simulink model "Non_ideal"  (R2025b)
settings: Solver=VariableStepAuto  StartTime=0.0  StopTime=4.6  RelTol=1e-3
values from neighbouring files (symbols this model uses):
  A0 = 1/w    (= 7.8125e-09)    [init.m]
  a1 = a(1)    [init.m]
  a2 = a(2)    [init.m]
  a3 = a(3)    [init.m]
  a4 = a(4)    [init.m]
  A_flick = 1e-9    (= 1e-09)    [init.m]
  Ain = 1.8    [init.m]
  Amax = 1.8    [init.m]
  b1 = b(1)    [init.m]
  c1 = c(1)    [init.m]
  c2 = c(2)    [init.m]
  c3 = c(3)    [init.m]
  c4 = c(4)    [init.m]
  fin = 250    [init.m]
  fir_coefficients = firpm(MaxTaps-1, F, A, W)    [fir_coeff.m]
  fs = 128e3    (= 128000)    [init.m]
  fsr = (2*pi)*fs*1.8    (= 1447645.89477)    [init.m]
  g1 = g(1)    [init.m]
  g2 = g(2)    [init.m]
  Gj = 1e5    (= 100000)    [init.m]
  h = h / max(h)    [cic_comp_coeff_calc.m]    (also in gain_calculate.m = tf.k * evalRP(tf.zeros,z) ./ evalRP(tf.poles,z))
  halfband_coeff = firhalfband(N, kaiser(N+1, beta))    [fir_halfband_coeff.m]
  j_rms = 0.3    [init.m]
  scale = 1.6    [init.m]
  w = (2*(1:order)'-1)*pi/order    [gain_calculate.m]    (also in init.m = 128000000)
libraries: dsphdlfiltering2 x4, dspsigops x2, dspfdesign x1
settings Model: Creator=sohom  LastModifiedBy=dhruv

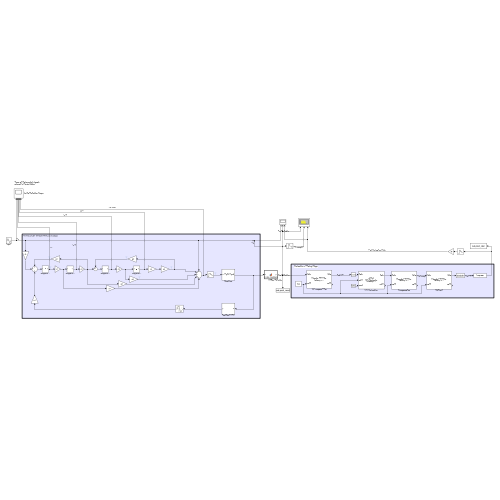
[thumbnail: Simulink's stored preview of the top-level diagram]
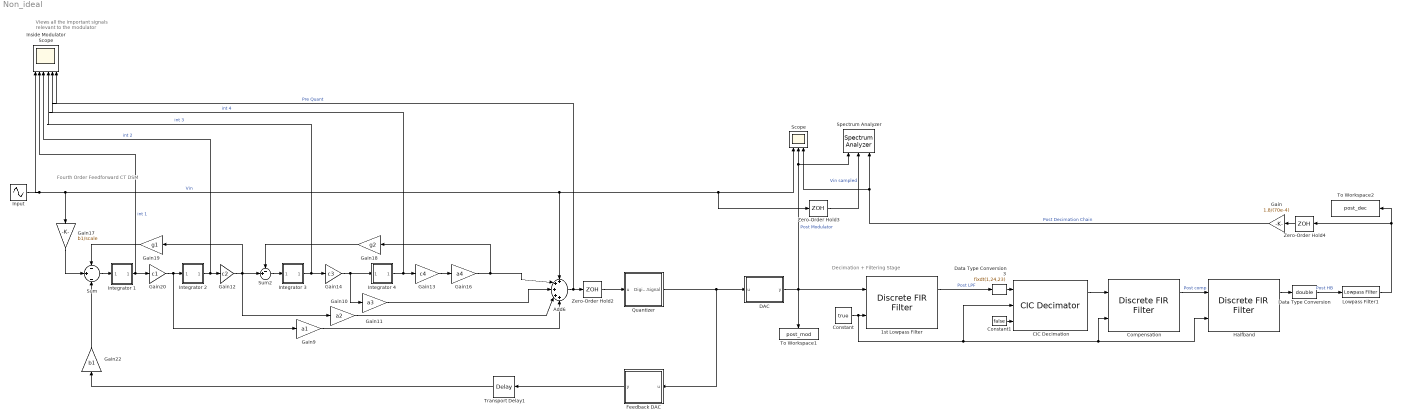
== system Non_ideal ==
  note: Fourth Order Feedforward CT DSM
  note: Views all the important signals
      | relevant to the modulator
  note: Decimation + Filtering Stage
  1st Lowpass Filter : dsphdlfiltering2/Discrete FIR Filter  NumeratorSource=Property  Numerator=[fir_coefficients]  NumeratorPrototype=[]  FilterStructure=Direct form systolic  SerializationOption=Minimum number of cycles between valid input samples  NumCycles=2  NumberOfMultipliers=2  SimulateUsing=Code generation  roundingMode=Floor  overflowMode=off  CoefficientsDataTypeStr=Inherit: Same word length as input  ResetInputPort=off  HDLGlobalReset=off  CoeffMultiplier=Multiplier  UseMultForPow2Coeff=on  FrameInputSymmOptim=on
  Add6 : Sum  Inputs=+++++
  CIC Decimation : dsphdlfiltering2/CIC Decimator  DecimationSource=Property  DecimationFactor=32  MaxDecimationFactor=2  DifferentialDelay=1  NumSections=5  GainCorrection=on  SimulateUsing=Code generation  OutputDataType=Full precision  OutputWordLength=16  ResetInputPort=on  HDLGlobalReset=off
  Compensation : dsphdlfiltering2/Discrete FIR Filter  NumeratorSource=Property  Numerator=[h]  NumeratorPrototype=[]  FilterStructure=Direct form systolic  SerializationOption=Minimum number of cycles between valid input samples  NumCycles=2  NumberOfMultipliers=2  SimulateUsing=Code generation  roundingMode=Floor  overflowMode=off  CoefficientsDataTypeStr=Inherit: Same word length as input  ResetInputPort=off  HDLGlobalReset=off  CoeffMultiplier=Multiplier  UseMultForPow2Coeff=on  FrameInputSymmOptim=on
  Constant : Constant  Value=true
  Constant1 : Constant  Value=false
  DAC : MATLAB Function  TreatAsAtomicUnit=on
  Data Type Conversion : DataTypeConversion  OutDataTypeStr=double  RndMeth=Nearest  SaturateOnIntegerOverflow=off
  Data Type Conversion3 : DataTypeConversion  OutDataTypeStr=fixdt(1,24,23)  RndMeth=Nearest  SaturateOnIntegerOverflow=off
  Feedback DAC : Subsystem
  Gain : Gain  Gain=1.8/(70e-4)
  Gain10 : Gain  Gain=a2
  Gain11 : Gain  Gain=a3
  Gain12 : Gain  Gain=c2
  Gain13 : Gain  Gain=c4
  Gain14 : Gain  Gain=c3
  Gain16 : Gain  Gain=a4
  Gain17 : Gain  Gain=b1/scale
  Gain18 : Gain  Gain=g2
  Gain19 : Gain  Gain=g1
  Gain20 : Gain  Gain=c1
  Gain22 : Gain  Gain=b1
  Gain9 : Gain  Gain=a1
  Halfband : dsphdlfiltering2/Discrete FIR Filter  NumeratorSource=Property  Numerator=[halfband_coeff]  NumeratorPrototype=[]  FilterStructure=Direct form systolic  SerializationOption=Minimum number of cycles between valid input samples  NumCycles=2  NumberOfMultipliers=2  SimulateUsing=Code generation  roundingMode=Floor  overflowMode=off  CoefficientsDataTypeStr=Inherit: Same word length as input  ResetInputPort=off  HDLGlobalReset=off  CoeffMultiplier=Multiplier  UseMultForPow2Coeff=on  FrameInputSymmOptim=on
  Input : Sin  Amplitude=Ain  Frequency=2*pi*fin  SampleTime=0
  Inside Modulator Scope : Scope  NumInputPorts=6
      settings: ActiveDisplayYMinimum=-1  ActiveDisplayYMaximum=1  DataLoggingVariableName=ScopeData2
  Integrator 1 : Subsystem
      mask Display: image('download.png');
  Integrator 2 : Subsystem
      mask Display: image('download.png');
  Integrator 3 : Subsystem
      mask Display: image('download.png');
  Integrator 4 : Subsystem
      mask Display: image('download.png');
  Lowpass Filter1 : dspfdesign/Lowpass Filter  FilterType=FIR  DesignForMinimumOrder=on  FilterOrder=50  PassbandFrequency=1000  StopbandFrequency=2000  PassbandRipple=0.01  StopbandAttenuation=80  SampleRateMode=Specify on dialog  SampleRate=fs  SimulateUsing=Interpreted execution  roundingMode=Floor  coeffsDataTypeStr=fixdt(1,16)
  Quantizer : Subsystem
  Scope : Scope  NumInputPorts=3
      settings: ActiveDisplayYMinimum=-2.2360659087505561  ActiveDisplayYMaximum=2.257708308181404
  Spectrum Analyzer : SpectrumAnalyzer  NumInputPorts=3  WindowPosition=[0.000000,36.000000,1920.000000,1009.000000,]  ScopeFrameLocation=window  SampleRate=44.1e3  PlotAsTwoSidedSpectrum=off  WindowInvariantSamplesPerUpdate=on  FrequencySpan=Start and stop frequencies  StartFrequency=20  StopFrequency=20e3  YLimits=[NaN NaN]  ShowLegend=on  SelectedToolstripTab=spectrumAnalyzerToolstrip.measurementsTab
  Sum : Sum  Inputs=-|+|-
  Sum2 : Sum  Inputs=-+|
  To Workspace1 : ToWorkspace  VariableName=post_mod  SaveFormat=Timeseries  SampleTime=-1
  To Workspace2 : ToWorkspace  VariableName=post_dec  SaveFormat=Timeseries  SampleTime=-1
  Transport Delay1 : TransportDelay  DelayTime=0.1/fs
  Zero-Order Hold2 : ZeroOrderHold  SampleTime=1/fs
  Zero-Order Hold3 : ZeroOrderHold  SampleTime=1/fs
  Zero-Order Hold4 : ZeroOrderHold  SampleTime=1/fs
  wires:
  Gain11/1 -> Add6/3
  Gain10/1 -> Add6/4
  Gain17/1 -> Sum/2
  Gain22/1 -> Sum/3
  Gain19/1 -> Sum/1
  Gain16/1 -> Gain18/1, Add6/2
  Transport Delay1/1 -> Gain22/1
  Gain9/1 -> Add6/5
  Gain18/1 -> Sum2/1
  Gain12/1 -> Gain19/1, Sum2/2, Gain10/1
  Gain20/1 -> Integrator 2/1(Input), Gain9/1
  Gain14/1 -> Integrator 4/1(Input), Gain11/1
  Quantizer/1(Digital Signal) -> Feedback DAC/1(u), DAC/1(u)
  Zero-Order Hold2/1 -> Quantizer/1(u)
  Feedback DAC/1(y) -> Transport Delay1/1
  Sum/1 -> Integrator 1/1(Input)
  Sum2/1 -> Integrator 3/1(Input)
  Integrator 2/1(Output) -> Inside Modulator Scope/3, Gain12/1  "int 2"
  Integrator 4/1(Output) -> Gain13/1, Inside Modulator Scope/5  "int 4"
  Integrator 1/1(Output) -> Gain20/1, Inside Modulator Scope/2  "int 1"
  Add6/1 -> Inside Modulator Scope/6, Zero-Order Hold2/1  "Pre Quant"
  Integrator 3/1(Output) -> Inside Modulator Scope/4, Gain14/1  "int 3"
  Data Type Conversion/1 -> Lowpass Filter1/1  "Post HB"
  Compensation/1 -> Halfband/1  "Post comp"
  CIC Decimation/1 -> Compensation/1
  Zero-Order Hold4/1 -> Gain/1
  Halfband/1 -> Data Type Conversion/1
  Constant1/1 -> CIC Decimation/3
  DAC/1(y) -> Spectrum Analyzer/1, Scope/2, To Workspace1/1, 1st Lowpass Filter/1  "Post Modulator"
  Input/1 -> Inside Modulator Scope/1, Gain17/1, Zero-Order Hold3/1, Scope/1, Add6/1  "Vin"
  1st Lowpass Filter/1 -> Data Type Conversion3/1  "Post LPF"
  Lowpass Filter1/1 -> To Workspace2/1, Zero-Order Hold4/1
  Constant/1 -> CIC Decimation/2, Halfband/2, Compensation/2, 1st Lowpass Filter/2
  Zero-Order Hold3/1 -> Spectrum Analyzer/2  "Vin sampled"
  Data Type Conversion3/1 -> CIC Decimation/1
  Gain/1 -> Scope/3, Spectrum Analyzer/3  "Post Decimation Chain"
  Gain13/1 -> Gain16/1

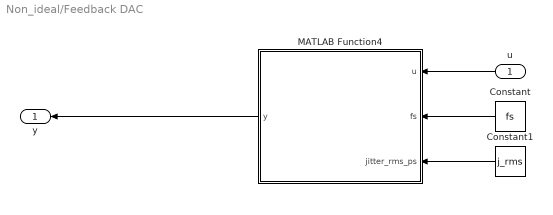
== system Non_ideal/Feedback DAC ==
  u : Inport
  Constant : Constant  Value=fs
  Constant1 : Constant  Value=j_rms
  MATLAB Function4 : MATLAB Function  TreatAsAtomicUnit=on
  y : Outport
  wires:
  MATLAB Function4/1(y) -> y/1
  Constant1/1 -> MATLAB Function4/3(jitter_rms_ps)
  Constant/1 -> MATLAB Function4/2(fs)
  u/1 -> MATLAB Function4/1(u)

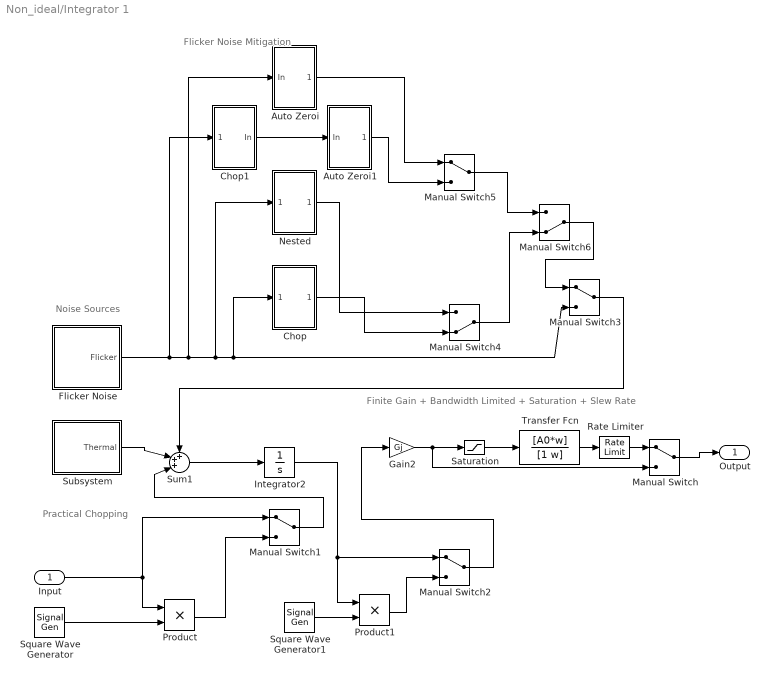
== system Non_ideal/Integrator 1 ==
  note: Finite Gain + Bandwidth Limited + Saturation + Slew Rate
  note: Flicker Noise Mitigation
  note: Practical Chopping
  note: Noise Sources
  Input : Inport
  Auto Zeroi : Subsystem
  Auto Zeroi1 : Subsystem
  Chop : Subsystem
  Chop1 : Subsystem
  Flicker Noise : Subsystem
  Gain2 : Gain  Gain=Gj
  Integrator2 : Integrator
  Manual Switch{,1..3,5} (5 alike) : ManualSwitch
  Manual Switch4 : ManualSwitch  CurrentSetting=0
  Manual Switch6 : ManualSwitch  CurrentSetting=0
  Nested : Subsystem
  Product : Product
  Product1 : Product
  Rate Limiter : RateLimiter  RisingSlewLimit=fsr  FallingSlewLimit=-fsr  SampleTimeMode=inherited
  Saturation : Saturate  UpperLimit=Amax  LowerLimit=-Amax
  Square Wave Generator : SignalGenerator  WaveForm=square  Frequency=8000
  Square Wave Generator1 : SignalGenerator  WaveForm=square  Frequency=8000
  Subsystem : Subsystem
  Sum1 : Sum  Inputs=+++|
  Transfer Fcn : TransferFcn  Numerator=[A0*w]  Denominator=[1 w]
  Output : Outport
  wires:
  Subsystem/1(Thermal) -> Sum1/2
  Manual Switch/1 -> Output/1
  Sum1/1 -> Integrator2/1
  Rate Limiter/1 -> Manual Switch/1
  Transfer Fcn/1 -> Rate Limiter/1
  Gain2/1 -> Manual Switch/2, Saturation/1
  Saturation/1 -> Transfer Fcn/1
  Square Wave Generator/1 -> Product/2
  Product/1 -> Manual Switch1/2
  Input/1 -> Manual Switch1/1, Product/1
  Product1/1 -> Manual Switch2/2
  Integrator2/1 -> Manual Switch2/1, Product1/1
  Square Wave Generator1/1 -> Product1/2
  Manual Switch2/1 -> Gain2/1
  Manual Switch1/1 -> Sum1/3
  Flicker Noise/1(Flicker) -> Chop1/1(Flicker), Auto Zeroi/1(In), Chop/1(Flicker), Manual Switch3/2, Nested/1(In1)
  Manual Switch3/1 -> Sum1/1
  Auto Zeroi/1(Out1) -> Manual Switch5/1
  Chop/1(Out1) -> Manual Switch4/2
  Nested/1(Out1) -> Manual Switch4/1
  Manual Switch4/1 -> Manual Switch6/2
  Manual Switch6/1 -> Manual Switch3/1
  Chop1/1(In) -> Auto Zeroi1/1(In)
  Auto Zeroi1/1(Out1) -> Manual Switch5/2
  Manual Switch5/1 -> Manual Switch6/1

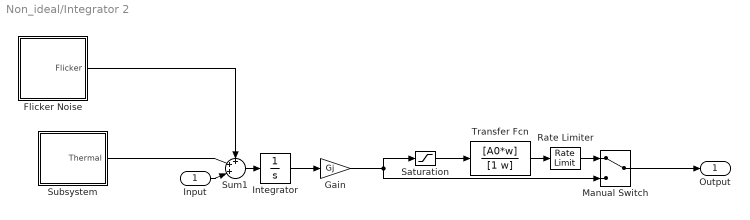
== system Non_ideal/Integrator 2 ==
  Input : Inport
  Flicker Noise : Subsystem
  Gain : Gain  Gain=Gj
  Integrator : Integrator
  Manual Switch : ManualSwitch
  Rate Limiter : RateLimiter  RisingSlewLimit=fsr  FallingSlewLimit=-fsr  SampleTimeMode=inherited
  Saturation : Saturate  UpperLimit=Amax  LowerLimit=-Amax
  Subsystem : Subsystem
  Sum1 : Sum  Inputs=+++|
  Transfer Fcn : TransferFcn  Numerator=[A0*w]  Denominator=[1 w]
  Output : Outport
  wires:
  Input/1 -> Sum1/3
  Subsystem/1(Thermal) -> Sum1/2
  Flicker Noise/1(Flicker) -> Sum1/1
  Manual Switch/1 -> Output/1
  Sum1/1 -> Integrator/1
  Integrator/1 -> Gain/1
  Rate Limiter/1 -> Manual Switch/1
  Transfer Fcn/1 -> Rate Limiter/1
  Gain/1 -> Manual Switch/2, Saturation/1
  Saturation/1 -> Transfer Fcn/1

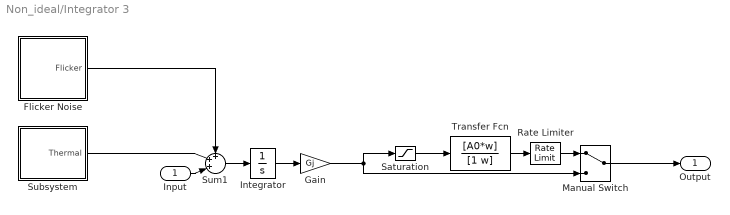
== system Non_ideal/Integrator 3 ==
  Input : Inport
  Flicker Noise : Subsystem
  Gain : Gain  Gain=Gj
  Integrator : Integrator
  Manual Switch : ManualSwitch
  Rate Limiter : RateLimiter  RisingSlewLimit=fsr  FallingSlewLimit=-fsr  SampleTimeMode=inherited
  Saturation : Saturate  UpperLimit=Amax  LowerLimit=-Amax
  Subsystem : Subsystem
  Sum1 : Sum  Inputs=+++|
  Transfer Fcn : TransferFcn  Numerator=[A0*w]  Denominator=[1 w]
  Output : Outport
  wires:
  Input/1 -> Sum1/3
  Subsystem/1(Thermal) -> Sum1/2
  Flicker Noise/1(Flicker) -> Sum1/1
  Manual Switch/1 -> Output/1
  Sum1/1 -> Integrator/1
  Integrator/1 -> Gain/1
  Rate Limiter/1 -> Manual Switch/1
  Transfer Fcn/1 -> Rate Limiter/1
  Gain/1 -> Manual Switch/2, Saturation/1
  Saturation/1 -> Transfer Fcn/1

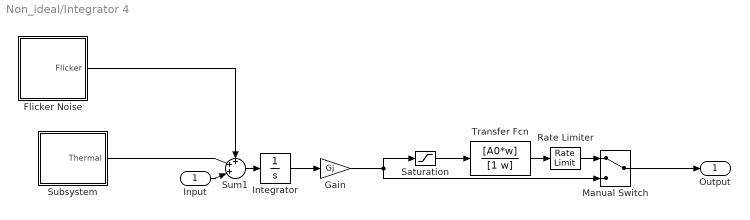
== system Non_ideal/Integrator 4 ==
  Input : Inport
  Flicker Noise : Subsystem
  Gain : Gain  Gain=Gj
  Integrator : Integrator
  Manual Switch : ManualSwitch
  Rate Limiter : RateLimiter  RisingSlewLimit=fsr  FallingSlewLimit=-fsr  SampleTimeMode=inherited
  Saturation : Saturate  UpperLimit=Amax  LowerLimit=-Amax
  Subsystem : Subsystem
  Sum1 : Sum  Inputs=+++|
  Transfer Fcn : TransferFcn  Numerator=[A0*w]  Denominator=[1 w]
  Output : Outport
  wires:
  Input/1 -> Sum1/3
  Subsystem/1(Thermal) -> Sum1/2
  Flicker Noise/1(Flicker) -> Sum1/1
  Manual Switch/1 -> Output/1
  Sum1/1 -> Integrator/1
  Integrator/1 -> Gain/1
  Rate Limiter/1 -> Manual Switch/1
  Transfer Fcn/1 -> Rate Limiter/1
  Gain/1 -> Manual Switch/2, Saturation/1
  Saturation/1 -> Transfer Fcn/1

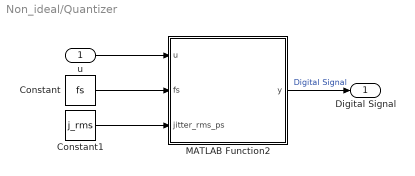
== system Non_ideal/Quantizer ==
  u : Inport
  Constant : Constant  Value=fs
  Constant1 : Constant  Value=j_rms
  MATLAB Function2 : MATLAB Function  TreatAsAtomicUnit=on
  Digital Signal : Outport
  wires:
  MATLAB Function2/1(y) -> Digital Signal/1  "Digital Signal"
  u/1 -> MATLAB Function2/1(u)
  Constant1/1 -> MATLAB Function2/3(jitter_rms_ps)
  Constant/1 -> MATLAB Function2/2(fs)

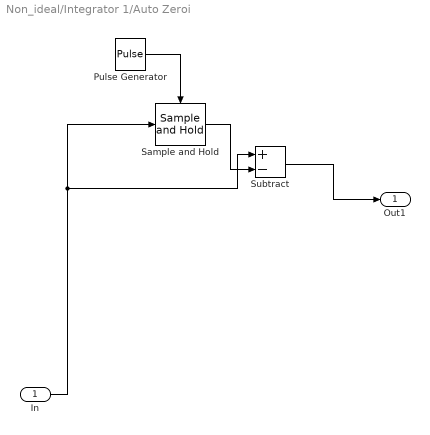
== system Non_ideal/Integrator 1/Auto Zeroi ==
  In : Inport
  Pulse Generator : DiscretePulseGenerator  PulseType=Time based  Period=10/128000
  Sample and Hold : dspsigops/Sample and Hold  trig=Rising edge  initCond=0  latchinput=off
  Subtract : Sum  Inputs=+-
  Out1 : Outport
  wires:
  Subtract/1 -> Out1/1
  Pulse Generator/1 -> Sample and Hold/Trigger
  In/1 -> Subtract/1, Sample and Hold/1
  Sample and Hold/1 -> Subtract/2

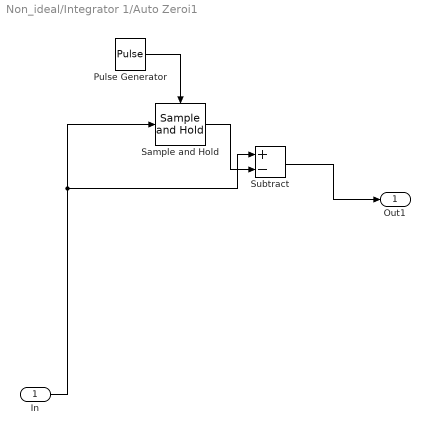
== system Non_ideal/Integrator 1/Auto Zeroi1 ==
  In : Inport
  Pulse Generator : DiscretePulseGenerator  PulseType=Time based  Period=10/128000
  Sample and Hold : dspsigops/Sample and Hold  trig=Rising edge  initCond=0  latchinput=off
  Subtract : Sum  Inputs=+-
  Out1 : Outport
  wires:
  Subtract/1 -> Out1/1
  Pulse Generator/1 -> Sample and Hold/Trigger
  In/1 -> Subtract/1, Sample and Hold/1
  Sample and Hold/1 -> Subtract/2

== system Non_ideal/Integrator 1/Chop ==
  Flicker : Inport
  Product3 : Product
  Square Wave Generator3 : SignalGenerator  WaveForm=square  Frequency=32000
  Out1 : Outport
  wires:
  Product3/1 -> Out1/1
  Square Wave Generator3/1 -> Product3/2
  Flicker/1 -> Product3/1

== system Non_ideal/Integrator 1/Chop1 ==
  Flicker : Inport
  Product3 : Product
  Square Wave Generator3 : SignalGenerator  WaveForm=square  Frequency=32000
  In : Outport
  wires:
  Product3/1 -> In/1
  Square Wave Generator3/1 -> Product3/2
  Flicker/1 -> Product3/1

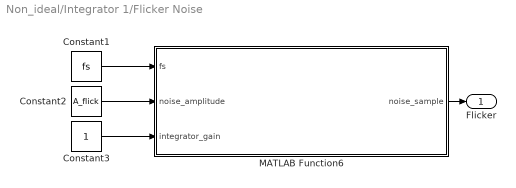
== system Non_ideal/Integrator 1/Flicker Noise ==
  Constant1 : Constant  Value=fs
  Constant2 : Constant  Value=A_flick
  Constant3 : Constant
  MATLAB Function6 : MATLAB Function  TreatAsAtomicUnit=on
  Flicker : Outport
  wires:
  Constant2/1 -> MATLAB Function6/2(noise_amplitude)
  Constant3/1 -> MATLAB Function6/3(integrator_gain)
  Constant1/1 -> MATLAB Function6/1(fs)
  MATLAB Function6/1(noise_sample) -> Flicker/1

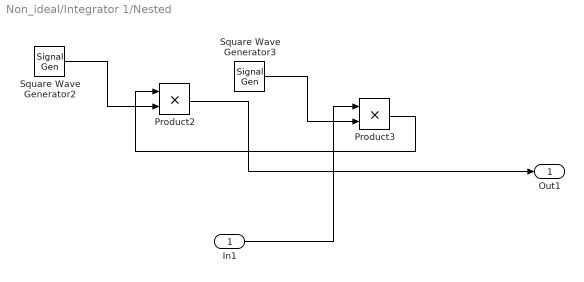
== system Non_ideal/Integrator 1/Nested ==
  In1 : Inport
  Product2 : Product
  Product3 : Product
  Square Wave Generator2 : SignalGenerator  WaveForm=square  Frequency=4000
  Square Wave Generator3 : SignalGenerator  WaveForm=square  Frequency=32000
  Out1 : Outport
  wires:
  Product2/1 -> Out1/1
  Square Wave Generator3/1 -> Product3/2
  Product3/1 -> Product2/1
  In1/1 -> Product3/1
  Square Wave Generator2/1 -> Product2/2

== system Non_ideal/Integrator 1/Subsystem ==
  Constant1 : Constant  Value=fs
  MATLAB Function6 : MATLAB Function  TreatAsAtomicUnit=on
  Thermal : Outport
  wires:
  Constant1/1 -> MATLAB Function6/1(fs)
  MATLAB Function6/1(noise_out) -> Thermal/1

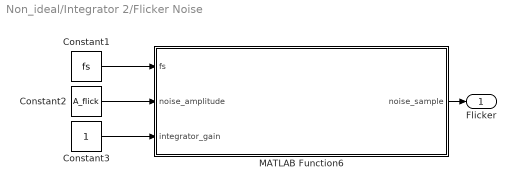
== system Non_ideal/Integrator 2/Flicker Noise ==
  Constant1 : Constant  Value=fs
  Constant2 : Constant  Value=A_flick
  Constant3 : Constant
  MATLAB Function6 : MATLAB Function  TreatAsAtomicUnit=on
  Flicker : Outport
  wires:
  Constant2/1 -> MATLAB Function6/2(noise_amplitude)
  Constant3/1 -> MATLAB Function6/3(integrator_gain)
  Constant1/1 -> MATLAB Function6/1(fs)
  MATLAB Function6/1(noise_sample) -> Flicker/1

== system Non_ideal/Integrator 2/Subsystem ==
  Constant1 : Constant  Value=fs
  MATLAB Function6 : MATLAB Function  TreatAsAtomicUnit=on
  Thermal : Outport
  wires:
  Constant1/1 -> MATLAB Function6/1(fs)
  MATLAB Function6/1(noise_out) -> Thermal/1

== system Non_ideal/Integrator 3/Flicker Noise ==
  Constant1 : Constant  Value=fs
  Constant2 : Constant  Value=A_flick
  Constant3 : Constant
  MATLAB Function6 : MATLAB Function  TreatAsAtomicUnit=on
  Flicker : Outport
  wires:
  Constant2/1 -> MATLAB Function6/2(noise_amplitude)
  Constant3/1 -> MATLAB Function6/3(integrator_gain)
  Constant1/1 -> MATLAB Function6/1(fs)
  MATLAB Function6/1(noise_sample) -> Flicker/1

== system Non_ideal/Integrator 3/Subsystem ==
  Constant1 : Constant  Value=fs
  MATLAB Function6 : MATLAB Function  TreatAsAtomicUnit=on
  Thermal : Outport
  wires:
  Constant1/1 -> MATLAB Function6/1(fs)
  MATLAB Function6/1(noise_out) -> Thermal/1

== system Non_ideal/Integrator 4/Flicker Noise ==
  Constant1 : Constant  Value=fs
  Constant2 : Constant  Value=A_flick
  Constant3 : Constant
  MATLAB Function6 : MATLAB Function  TreatAsAtomicUnit=on
  Flicker : Outport
  wires:
  Constant2/1 -> MATLAB Function6/2(noise_amplitude)
  Constant3/1 -> MATLAB Function6/3(integrator_gain)
  Constant1/1 -> MATLAB Function6/1(fs)
  MATLAB Function6/1(noise_sample) -> Flicker/1

== system Non_ideal/Integrator 4/Subsystem ==
  Constant1 : Constant  Value=fs
  MATLAB Function6 : MATLAB Function  TreatAsAtomicUnit=on
  Thermal : Outport
  wires:
  Constant1/1 -> MATLAB Function6/1(fs)
  MATLAB Function6/1(noise_out) -> Thermal/1

== matlab function Non_ideal/Integrator 2/Flicker Noise/MATLAB Function6 ==
  data: noise_sample output; fs input; noise_amplitude input; integrator_gain input
function noise_sample = flicker_noise_stream(fs, noise_amplitude, integrator_gain)
% 1/f Flicker Noise Generator for CTDSM
% Paste this entire function into Simulink MATLAB Function block
%
% Inputs:
%   fs               - Sampling frequency (Hz)
%   noise_amplitude  - Noise amplitude (V/sqrt(Hz) at 1Hz), e.g., 1e-7
%   integrator_gain  - Integrator coefficient, e.g., 1.0
%
% Output:
%   noise_sample     - Single noise sample for this time step

persistent generators counters num_gen

% Initialize on first call
if isempty(generators)
    num_gen = 16;
    generators = randn(num_gen, 1);
    counters = zeros(num_gen, 1);
end

% Generate 1/f noise using Voss-McCartney algorithm
noise_sample = 0;
for k = 1:num_gen
    counters(k) = counters(k) + 1;
    update_rate = 2^k;
    
    % Update generator when counter reaches update rate
    if counters(k) >= update_rate
        generators(k) = randn();
        counters(k) = 0;
    end
    
    noise_sample = noise_sample + generators(k);
end

% Normalize and scale
noise_sample = noise_sample / sqrt(num_gen);

% Scale with signal bandwidth (0.25 to 1 kHz)
signal_bw = 1000;
noise_sample = noise_sample * sqrt(signal_bw);

% Apply user-specified amplitude
noise_sample = noise_sample * noise_amplitude;

% Scale by integrator characteristics
noise_sample = noise_sample * sqrt(abs(integrator_gain));

% Convert from PSD to time-domain amplitude
noise_sample = noise_sample * sqrt(fs/2);

end

== matlab function Non_ideal/Integrator 1/Flicker Noise/MATLAB Function6 ==
  data: noise_sample output; fs input; noise_amplitude input; integrator_gain input
function noise_sample = flicker_noise_stream(fs, noise_amplitude, integrator_gain)
% 1/f Flicker Noise Generator for CTDSM
% Paste this entire function into Simulink MATLAB Function block
%
% Inputs:
%   fs               - Sampling frequency (Hz)
%   noise_amplitude  - Noise amplitude (V/sqrt(Hz) at 1Hz), e.g., 1e-7
%   integrator_gain  - Integrator coefficient, e.g., 1.0
%
% Output:
%   noise_sample     - Single noise sample for this time step

persistent generators counters num_gen

% Initialize on first call
if isempty(generators)
    num_gen = 16;
    generators = randn(num_gen, 1);
    counters = zeros(num_gen, 1);
end

% Generate 1/f noise using Voss-McCartney algorithm
noise_sample = 0;
for k = 1:num_gen
    counters(k) = counters(k) + 1;
    update_rate = 2^k;
    
    % Update generator when counter reaches update rate
    if counters(k) >= update_rate
        generators(k) = randn();
        counters(k) = 0;
    end
    
    noise_sample = noise_sample + generators(k);
end

% Normalize and scale
noise_sample = noise_sample / sqrt(num_gen);

% Scale with signal bandwidth (0.25 to 1 kHz)
signal_bw = 1000;
noise_sample = noise_sample * sqrt(signal_bw);

% Apply user-specified amplitude
noise_sample = noise_sample * noise_amplitude;

% Scale by integrator characteristics
noise_sample = noise_sample * sqrt(abs(integrator_gain));

% Convert from PSD to time-domain amplitude
noise_sample = noise_sample * sqrt(fs/2);

end

== matlab function Non_ideal/Quantizer/MATLAB Function2 ==
  data: u input; y output; fs input; jitter_rms_ps input
function y = ct_quantizer(u, fs, jitter_rms_ps)
% CT DSM Quantizer with Clock Jitter and Thermometer Code Output
% Insert this as a MATLAB Function block in Simulink
%
% INPUTS:
%   u              - Input signal from loop filter
%   fs             - Sampling frequency (Hz)
%   jitter_rms_ps  - RMS clock jitter in picoseconds (ps)
%                    Set to 0 for ideal case (no jitter)
%
% PARAMETERS (modify these at the top)
% =========================================================================
N_LEVELS = 16;           % Number of quantization levels (1-bit = 2 levels)
INPUT_MIN = -1.8;        % Minimum input range (V)
INPUT_MAX = 1.8;         % Maximum input range (V)

% PERSISTENT VARIABLES - MUST BE DECLARED AT TOP!
% =========================================================================
persistent u_prev;

% JITTER GUIDELINES (typical values for different applications):
% =========================================================================
% Ultra-low jitter (< 100 fs):   20+ bit ENOB, high-end audio/instrumentation
% Low jitter (100 fs - 1 ps):    18-20 bit ENOB, precision converters
% Moderate jitter (1-10 ps):     14-16 bit ENOB, general purpose ADCs
% High jitter (10-100 ps):       10-12 bit ENOB, cost-optimized designs
% Very high jitter (> 100 ps):   < 10 bit ENOB, low-performance systems
%
% For YOUR CTDSM (ENOB 16-19 target):
% RECOMMENDED: jitter_rms_ps = 0.5 to 2 ps (500 fs to 2 ps)
%
% Jitter SNR Formula: SNR_jitter(dB) = -20*log10(2*pi*f_in*σ_jitter)
% For f_in = 1 kHz, jitter = 1 ps: SNR ≈ 104 dB (17 bits)
% =========================================================================

% Validate parameters
assert(N_LEVELS >= 2, 'N_LEVELS must be at least 2');
assert(INPUT_MAX > INPUT_MIN, 'INPUT_MAX must be greater than INPUT_MIN');
assert(fs > 0, 'Sampling frequency must be positive');
assert(jitter_rms_ps >= 0, 'Jitter must be non-negative');

% Initialize persistent variable on first call
if isempty(u_prev)
    u_prev = u;
end

% Calculate jitter-induced timing error
if jitter_rms_ps > 0
    % Convert jitter from picoseconds to seconds
    jitter_rms_sec = jitter_rms_ps * 1e-12;
    
    % Generate random timing error (Gaussian distribution)
    timing_error = jitter_rms_sec * randn();
    
    % Calculate slew rate
    Ts = 1/fs;  % Sampling period
    slew_rate = (u - u_prev) / Ts;  % V/s
    
    % Calculate voltage error due to timing jitter
    % ΔV = (dV/dt) × Δt
    voltage_error = slew_rate * timing_error;
    
    % Apply jitter error to input
    u_jittered = u + voltage_error;
else
    % Ideal case: no jitter
    u_jittered = u;
end

% Update previous value for next iteration
u_prev = u;

% Input saturation (clip to range)
u_clipped = max(INPUT_MIN, min(INPUT_MAX, u_jittered));

% Mid-tread quantizer: zero is a quantization level
% For N levels, we have (N-1) thresholds
if N_LEVELS == 2
    % Special case: 1-bit quantizer
    % Threshold at 0 (mid-tread)
    if u_clipped >= 0
        quant_level = 1;  % Upper level
    else
        quant_level = 0;  % Lower level
    end
else
    % Multi-bit quantizer
    % Calculate thresholds for mid-tread configuration
    step = (INPUT_MAX - INPUT_MIN) / (N_LEVELS - 1);
    
    % Find which level the input corresponds to
    quant_level = round((u_clipped - INPUT_MIN) / step);
    
    % Ensure level is in valid range [0, N_LEVELS-1]
    quant_level = max(0, min(N_LEVELS - 1, quant_level));
end

% Convert to thermometer code
thermometer = zeros(1, N_LEVELS - 1);
for i = 1:(N_LEVELS - 1)
    if i <= quant_level
        thermometer(i) = 1;
    end
end

% Output as column vector
y = thermometer';

end

== matlab function Non_ideal/Integrator 2/Subsystem/MATLAB Function6 ==
  data: fs input; noise_out output
function noise_out = thermal_noise_circuit_based(fs)
    % Physical parameters
    T = 300;                    % Temperature (K)
    k = 1.38e-23;              % Boltzmann constant (J/K)
    
    % CIRCUIT PARAMETERS - These should come from your circuit design!
    % =================================================================
    
    % Option A: If you have op-amp specs
    % Input-referred noise voltage density (typical op-amp datasheet value)
    % Examples:
    %   - Precision op-amp: 5-10 nV/√Hz
    %   - General purpose: 10-20 nV/√Hz
    %   - Low noise: 1-5 nV/√Hz
    e_n = 10e-9;  % V/√Hz (10 nV/√Hz - typical precision op-amp)
    
    % Option B: If you have resistor values
    % Typical switched-capacitor or continuous-time integrator
    R_eq = 10e3;  % Equivalent noise resistance (10 kΩ typical)
    
    % Choose one method:
    % Method 1: Direct from op-amp noise spec
    noise_density = e_n;  % V/√Hz
    
    % Method 2: From thermal resistance
    % noise_density = sqrt(4 * k * T * R_eq);  % V/√Hz
    
    % =================================================================
    
    % Noise bandwidth (full Nyquist)
    BW = fs / 2;
    
    % Total RMS noise
    V_noise_rms = noise_density * sqrt(BW);
    
    % Generate white Gaussian noise sample
    % Scale to match power spectral density
    noise_out = V_noise_rms * randn();
    
end

== matlab function Non_ideal/Feedback DAC/MATLAB Function4 ==
  data: u input; y output; fs input; jitter_rms_ps input
function y = ct_dac_feedback(u, fs, jitter_rms_ps)
% CT DSM Feedback DAC with Clock Jitter - Converts Thermometer Code to Analog Level
% Insert this as a MATLAB Function block in Simulink
%
% INPUTS:
%   u              - Thermometer code from quantizer
%   fs             - Sampling frequency (Hz)
%   jitter_rms_ps  - RMS clock jitter in picoseconds (ps)
%                    Set to 0 for ideal case (no jitter)
%
% PARAMETERS (must match quantizer settings)
% =========================================================================
N_LEVELS = 16;           % Number of quantization levels (must match quantizer)
OUTPUT_MIN = -1.8;       % Minimum output voltage/amplitude (V)
OUTPUT_MAX = 1.8;        % Maximum output voltage/amplitude (V)

% PERSISTENT VARIABLES - MUST BE DECLARED AT TOP!
% =========================================================================
persistent y_prev;

% JITTER GUIDELINES FOR FEEDBACK DAC (MORE CRITICAL THAN QUANTIZER):
% =========================================================================
% The feedback DAC jitter is NOT noise-shaped and appears directly at input!
% DAC jitter requirements are typically 2-5x stricter than quantizer jitter.
%
% For CTDSM (ENOB 16-19 target):
% RECOMMENDED: jitter_rms_ps = 0.2 to 1 ps (200 fs to 1 ps)
% =========================================================================

% Validate parameters
assert(N_LEVELS >= 2, 'N_LEVELS must be at least 2');
assert(OUTPUT_MAX > OUTPUT_MIN, 'OUTPUT_MAX must be greater than OUTPUT_MIN');
assert(fs > 0, 'Sampling frequency must be positive');
assert(jitter_rms_ps >= 0, 'Jitter must be non-negative');

% Decode thermometer code to level
if N_LEVELS == 2
    % Special case: 1-bit (single element vector)
    level = u(1);  % 0 or 1
else
    % Multi-bit: count number of ones in thermometer code
    level = sum(u);  % Level from 0 to (N_LEVELS-1)
end

% Convert level to analog output (mid-tread)
if N_LEVELS == 2
    % 1-bit: simple bipolar mapping
    if level == 0
        y_ideal = OUTPUT_MIN;
    else
        y_ideal = OUTPUT_MAX;
    end
else
    % Multi-bit: linear mapping
    step = (OUTPUT_MAX - OUTPUT_MIN) / (N_LEVELS - 1);
    y_ideal = OUTPUT_MIN + level * step;
end

% Initialize persistent variable on first call
if isempty(y_prev)
    y_prev = y_ideal;
end

% Apply DAC clock jitter effects
if jitter_rms_ps > 0
    % Convert jitter from picoseconds to seconds
    jitter_rms_sec = jitter_rms_ps * 1e-12;
    
    % Generate random timing error (Gaussian distribution)
    timing_error = jitter_rms_sec * randn();
    
    % Calculate DAC output slew rate (how fast DAC is switching)
    Ts = 1/fs;  % Sampling period
    dac_slew_rate = (y_ideal - y_prev) / Ts;  % V/s
    
    % Voltage error due to timing jitter at DAC output
    % ΔV = (dV/dt) × Δt
    voltage_error = dac_slew_rate * timing_error;
    
    % Apply jitter error to DAC output
    y = y_ideal + voltage_error;
    
    % Optional: Add saturation to prevent unrealistic outputs
    y = max(OUTPUT_MIN, min(OUTPUT_MAX, y));
else
    % Ideal case: no jitter
    y = y_ideal;
end

% Update previous value for next iteration
y_prev = y_ideal;

end

== matlab function Non_ideal/DAC ==
  data: u input; y output
function y = ct_dac_feedback(u)
% CT DSM Feedback DAC - Converts Thermometer Code to Analog Level
% Insert this as a MATLAB Function block in Simulink
% Compatible with ct_quantizer output
%
% PARAMETERS (must match quantizer settings)
% =========================================================================
N_LEVELS = 16;           % Number of quantization levels (must match quantizer)
OUTPUT_MIN = -1.8;      % Minimum output voltage/amplitude
OUTPUT_MAX = 1.8;       % Maximum output voltage/amplitude
% =========================================================================

% Validate parameters
assert(N_LEVELS >= 2, 'N_LEVELS must be at least 2');
assert(OUTPUT_MAX > OUTPUT_MIN, 'OUTPUT_MAX must be greater than OUTPUT_MIN');

% Decode thermometer code to level
% Thermometer code has (N_LEVELS - 1) bits
% Count the number of ones to get the level
if N_LEVELS == 2
    % Special case: 1-bit (single element vector)
    % u is [0] or [1]
    level = u(1);  % 0 or 1
else
    % Multi-bit: count number of ones in thermometer code
    level = sum(u);  % This gives level from 0 to (N_LEVELS-1)
end

% Convert level to analog output (mid-tread)
% Map level [0, 1, 2, ..., N_LEVELS-1] to analog range
% For mid-tread, ensure level corresponds to actual output values
if N_LEVELS == 2
    % 1-bit: simple bipolar mapping
    % Level 0 -> OUTPUT_MIN (-1.8)
    % Level 1 -> OUTPUT_MAX (+1.8)
    if level == 0
        y = OUTPUT_MIN;
    else
        y = OUTPUT_MAX;
    end
else
    % Multi-bit: linear mapping
    % Map level to output range with mid-tread alignment
    step = (OUTPUT_MAX - OUTPUT_MIN) / (N_LEVELS - 1);
    y = OUTPUT_MIN + level * step;
end

end

% =========================================================================
% USAGE INSTRUCTIONS FOR SIMULINK:
% =========================================================================
% 1. Add a MATLAB Function block after your quantizer
% 2. Double-click the block and paste this entire code
% 3. Connect quantizer output (thermometer code) to this block's input
% 4. This block's output goes to the feedback path (summed with input)
%
% SIGNAL FLOW:
%   Input → [Σ] → Loop Filter → Quantizer → Output
%            ↑                      ↓
%            └──────── DAC ─────────┘
%
% For 2-level (1-bit):
%   Thermometer [0] → Analog output = -1.8
%   Thermometer [1] → Analog output = +1.8
%
% For 4-level (2-bit):
%   Thermometer [0 0 0] → -1.8
%   Thermometer [1 0 0] → -0.6
%   Thermometer [1 1 0] → +0.6
%   Thermometer [1 1 1] → +1.8
%
% NOTES:
% - N_LEVELS, OUTPUT_MIN, OUTPUT_MAX must match quantizer parameters
% - This is an ideal DAC (no delay, noise, or mismatch)
% - For CT-DSM, this typically runs continuously (no sample/hold needed)
% - Output is continuous-time analog signal fed back to input summer
% =========================================================================

== matlab function Non_ideal/Integrator 3/Flicker Noise/MATLAB Function6 ==
  data: noise_sample output; fs input; noise_amplitude input; integrator_gain input
function noise_sample = flicker_noise_stream(fs, noise_amplitude, integrator_gain)
% 1/f Flicker Noise Generator for CTDSM
% Paste this entire function into Simulink MATLAB Function block
%
% Inputs:
%   fs               - Sampling frequency (Hz)
%   noise_amplitude  - Noise amplitude (V/sqrt(Hz) at 1Hz), e.g., 1e-7
%   integrator_gain  - Integrator coefficient, e.g., 1.0
%
% Output:
%   noise_sample     - Single noise sample for this time step

persistent generators counters num_gen

% Initialize on first call
if isempty(generators)
    num_gen = 16;
    generators = randn(num_gen, 1);
    counters = zeros(num_gen, 1);
end

% Generate 1/f noise using Voss-McCartney algorithm
noise_sample = 0;
for k = 1:num_gen
    counters(k) = counters(k) + 1;
    update_rate = 2^k;
    
    % Update generator when counter reaches update rate
    if counters(k) >= update_rate
        generators(k) = randn();
        counters(k) = 0;
    end
    
    noise_sample = noise_sample + generators(k);
end

% Normalize and scale
noise_sample = noise_sample / sqrt(num_gen);

% Scale with signal bandwidth (0.25 to 1 kHz)
signal_bw = 1000;
noise_sample = noise_sample * sqrt(signal_bw);

% Apply user-specified amplitude
noise_sample = noise_sample * noise_amplitude;

% Scale by integrator characteristics
noise_sample = noise_sample * sqrt(abs(integrator_gain));

% Convert from PSD to time-domain amplitude
noise_sample = noise_sample * sqrt(fs/2);

end

== matlab function Non_ideal/Integrator 3/Subsystem/MATLAB Function6 ==
  data: fs input; noise_out output
function noise_out = thermal_noise_circuit_based(fs)
    % Physical parameters
    T = 300;                    % Temperature (K)
    k = 1.38e-23;              % Boltzmann constant (J/K)
    
    % CIRCUIT PARAMETERS - These should come from your circuit design!
    % =================================================================
    
    % Option A: If you have op-amp specs
    % Input-referred noise voltage density (typical op-amp datasheet value)
    % Examples:
    %   - Precision op-amp: 5-10 nV/√Hz
    %   - General purpose: 10-20 nV/√Hz
    %   - Low noise: 1-5 nV/√Hz
    e_n = 10e-9;  % V/√Hz (10 nV/√Hz - typical precision op-amp)
    
    % Option B: If you have resistor values
    % Typical switched-capacitor or continuous-time integrator
    R_eq = 10e3;  % Equivalent noise resistance (10 kΩ typical)
    
    % Choose one method:
    % Method 1: Direct from op-amp noise spec
    noise_density = e_n;  % V/√Hz
    
    % Method 2: From thermal resistance
    % noise_density = sqrt(4 * k * T * R_eq);  % V/√Hz
    
    % =================================================================
    
    % Noise bandwidth (full Nyquist)
    BW = fs / 2;
    
    % Total RMS noise
    V_noise_rms = noise_density * sqrt(BW);
    
    % Generate white Gaussian noise sample
    % Scale to match power spectral density
    noise_out = V_noise_rms * randn();
    
end

== matlab function Non_ideal/Integrator 4/Flicker Noise/MATLAB Function6 ==
  data: noise_sample output; fs input; noise_amplitude input; integrator_gain input
function noise_sample = flicker_noise_stream(fs, noise_amplitude, integrator_gain)
% 1/f Flicker Noise Generator for CTDSM
% Paste this entire function into Simulink MATLAB Function block
%
% Inputs:
%   fs               - Sampling frequency (Hz)
%   noise_amplitude  - Noise amplitude (V/sqrt(Hz) at 1Hz), e.g., 1e-7
%   integrator_gain  - Integrator coefficient, e.g., 1.0
%
% Output:
%   noise_sample     - Single noise sample for this time step

persistent generators counters num_gen

% Initialize on first call
if isempty(generators)
    num_gen = 16;
    generators = randn(num_gen, 1);
    counters = zeros(num_gen, 1);
end

% Generate 1/f noise using Voss-McCartney algorithm
noise_sample = 0;
for k = 1:num_gen
    counters(k) = counters(k) + 1;
    update_rate = 2^k;
    
    % Update generator when counter reaches update rate
    if counters(k) >= update_rate
        generators(k) = randn();
        counters(k) = 0;
    end
    
    noise_sample = noise_sample + generators(k);
end

% Normalize and scale
noise_sample = noise_sample / sqrt(num_gen);

% Scale with signal bandwidth (0.25 to 1 kHz)
signal_bw = 1000;
noise_sample = noise_sample * sqrt(signal_bw);

% Apply user-specified amplitude
noise_sample = noise_sample * noise_amplitude;

% Scale by integrator characteristics
noise_sample = noise_sample * sqrt(abs(integrator_gain));

% Convert from PSD to time-domain amplitude
noise_sample = noise_sample * sqrt(fs/2);

end

== matlab function Non_ideal/Integrator 4/Subsystem/MATLAB Function6 ==
  data: fs input; noise_out output
function noise_out = thermal_noise_circuit_based(fs)
    % Physical parameters
    T = 300;                    % Temperature (K)
    k = 1.38e-23;              % Boltzmann constant (J/K)
    
    % CIRCUIT PARAMETERS - These should come from your circuit design!
    % =================================================================
    
    % Option A: If you have op-amp specs
    % Input-referred noise voltage density (typical op-amp datasheet value)
    % Examples:
    %   - Precision op-amp: 5-10 nV/√Hz
    %   - General purpose: 10-20 nV/√Hz
    %   - Low noise: 1-5 nV/√Hz
    e_n = 10e-9;  % V/√Hz (10 nV/√Hz - typical precision op-amp)
    
    % Option B: If you have resistor values
    % Typical switched-capacitor or continuous-time integrator
    R_eq = 10e3;  % Equivalent noise resistance (10 kΩ typical)
    
    % Choose one method:
    % Method 1: Direct from op-amp noise spec
    noise_density = e_n;  % V/√Hz
    
    % Method 2: From thermal resistance
    % noise_density = sqrt(4 * k * T * R_eq);  % V/√Hz
    
    % =================================================================
    
    % Noise bandwidth (full Nyquist)
    BW = fs / 2;
    
    % Total RMS noise
    V_noise_rms = noise_density * sqrt(BW);
    
    % Generate white Gaussian noise sample
    % Scale to match power spectral density
    noise_out = V_noise_rms * randn();
    
end

== matlab function Non_ideal/Integrator 1/Subsystem/MATLAB Function6 ==
  data: fs input; noise_out output
function noise_out = thermal_noise_circuit_based(fs)
    % Physical parameters
    T = 300;                    % Temperature (K)
    k = 1.38e-23;              % Boltzmann constant (J/K)
    
    % CIRCUIT PARAMETERS - These should come from your circuit design!
    % =================================================================
    
    % Option A: If you have op-amp specs
    % Input-referred noise voltage density (typical op-amp datasheet value)
    % Examples:
    %   - Precision op-amp: 5-10 nV/√Hz
    %   - General purpose: 10-20 nV/√Hz
    %   - Low noise: 1-5 nV/√Hz
    e_n = 10e-9;  % V/√Hz (10 nV/√Hz - typical precision op-amp)
    
    % Option B: If you have resistor values
    % Typical switched-capacitor or continuous-time integrator
    R_eq = 10e3;  % Equivalent noise resistance (10 kΩ typical)
    
    % Choose one method:
    % Method 1: Direct from op-amp noise spec
    noise_density = e_n;  % V/√Hz
    
    % Method 2: From thermal resistance
    % noise_density = sqrt(4 * k * T * R_eq);  % V/√Hz
    
    % =================================================================
    
    % Noise bandwidth (full Nyquist)
    BW = fs / 2;
    
    % Total RMS noise
    V_noise_rms = noise_density * sqrt(BW);
    
    % Generate white Gaussian noise sample
    % Scale to match power spectral density
    noise_out = V_noise_rms * randn();
    
end
